simulink model "APP_SelSig"  (R2018a)
settings: configuration reference "cs_ert" (kept outside this file)
model workspace (MAT data in the model file):
  APP_SelSig_DT = 10
values from neighbouring files (symbols this model uses):
  APP_duLimErrPos_C = 1000.0    [APP_SelSig.sldd]
  APP_uAPPDef_C = 0.0    [APP_SelSig.sldd]
  APP_uRaw2Offset_C = 0.0    [APP_SelSig.sldd]
  MoFAPP_dRawSigFac_C = 2.0    [APP_SelSig.sldd]
libraries: simulink x1, sllib x1
settings Model: DataDictionary=APP_SelSig.sldd  Creator=zhoutinglin  LastModifiedBy=zhoutinglin

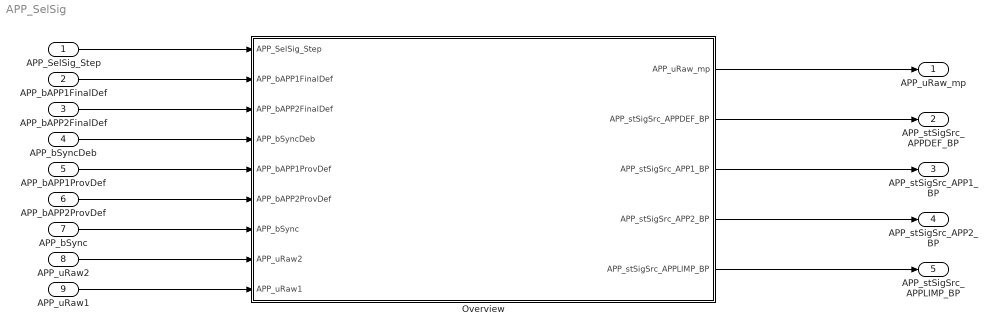
== system APP_SelSig ==
  APP_SelSig_Step : Inport  OutputFunctionCall=on
  APP_bAPP1FinalDef : Inport  Description=Status Sensor 1 of the acceleration pedal finally defect  Port=2  OutMin=0  OutMax=1  OutDataTypeStr=boolean  PortDimensions=[1 1]
  APP_bAPP2FinalDef : Inport  Description=Status Sensor 2 of the acceleration pedal finally defect  Port=3  OutMin=0  OutMax=1  OutDataTypeStr=boolean  PortDimensions=[1 1]
  APP_bSyncDeb : Inport  Description=Status debounced sync check  Port=4  OutMin=0  OutMax=1  OutDataTypeStr=boolean  PortDimensions=[1 1]
  APP_bAPP1ProvDef : Inport  Description=Status Sensor 1 of the acceleration pedal temporary defect  Port=5  OutMin=0  OutMax=1  OutDataTypeStr=boolean  PortDimensions=[1 1]
  APP_bAPP2ProvDef : Inport  Description=Status Sensor 2 of the acceleration pedal temporary defect  Port=6  OutMin=0  OutMax=1  OutDataTypeStr=boolean  PortDimensions=[1 1]
  APP_bSync : Inport  Description=Status temporary sync check  Port=7  OutMin=0  OutMax=1  OutDataTypeStr=boolean  PortDimensions=[1 1]
  APP_uRaw2 : Inport  Description=Acceleration Pedal Position E  Port=8  OutMin=0  OutMax=5000  OutDataTypeStr=Volt_mV  Unit=mv  PortDimensions=[1 1]
  APP_uRaw1 : Inport  Description=Acceleration Pedal Position D  Port=9  OutMin=0  OutMax=5000  OutDataTypeStr=Volt_mV  Unit=mv  PortDimensions=[1 1]
  Overview : Subsystem
  APP_uRaw_mp : Outport  Description=Acceleration pedal position raw value  OutMin=0  OutMax=5000  OutDataTypeStr=Volt_mV  Unit=mv  PortDimensions=[1 1]
  APP_stSigSrc_APPDEF_BP : Outport  Description=both the sensors are defective. Use the default value  Port=2  OutMin=0  OutMax=1  OutDataTypeStr=boolean  PortDimensions=[1 1]
  APP_stSigSrc_APP1_BP : Outport  Description=Sensor 1 is the reference variable, Sensor 2 value is defective  Port=3  OutMin=0  OutMax=1  OutDataTypeStr=boolean  PortDimensions=[1 1]
  APP_stSigSrc_APP2_BP : Outport  Description=Sensor 2 is the reference variable,Sensor1 value is defective  Port=4  OutMin=0  OutMax=1  OutDataTypeStr=boolean  PortDimensions=[1 1]
  APP_stSigSrc_APPLIMP_BP : Outport  Description=Substitute operation active, accelerator pedal sensor value and accelerator pedal sensor increase are limited  Port=5  OutMin=0  OutMax=1  OutDataTypeStr=boolean  PortDimensions=[1 1]
  wires:
  APP_SelSig_Step/1 -> Overview/1(APP_SelSig_Step)
  APP_bAPP1FinalDef/1 -> Overview/2(APP_bAPP1FinalDef)
  APP_bAPP2FinalDef/1 -> Overview/3(APP_bAPP2FinalDef)
  APP_bSyncDeb/1 -> Overview/4(APP_bSyncDeb)
  APP_bAPP1ProvDef/1 -> Overview/5(APP_bAPP1ProvDef)
  APP_bAPP2ProvDef/1 -> Overview/6(APP_bAPP2ProvDef)
  APP_bSync/1 -> Overview/7(APP_bSync)
  APP_uRaw2/1 -> Overview/8(APP_uRaw2)
  APP_uRaw1/1 -> Overview/9(APP_uRaw1)
  Overview/1(APP_uRaw_mp) -> APP_uRaw_mp/1
  Overview/2(APP_stSigSrc_APPDEF_BP) -> APP_stSigSrc_APPDEF_BP/1
  Overview/3(APP_stSigSrc_APP1_BP) -> APP_stSigSrc_APP1_BP/1
  Overview/4(APP_stSigSrc_APP2_BP) -> APP_stSigSrc_APP2_BP/1
  Overview/5(APP_stSigSrc_APPLIMP_BP) -> APP_stSigSrc_APPLIMP_BP/1

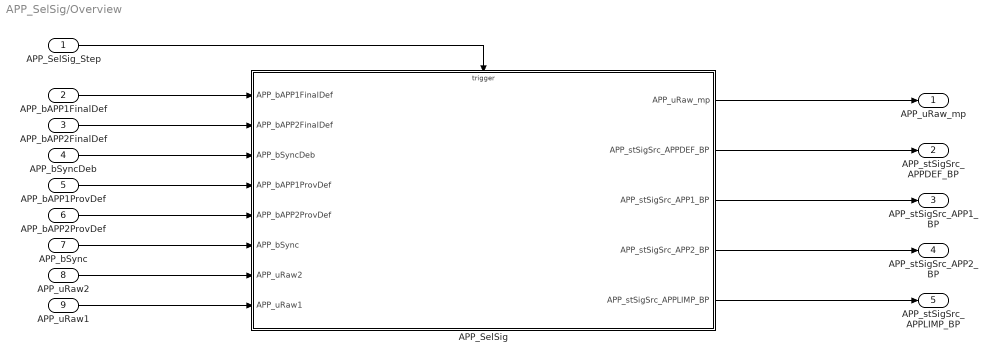
== system APP_SelSig/Overview ==
  APP_SelSig_Step : Inport
  APP_bAPP1FinalDef : Inport  Port=2
  APP_bAPP2FinalDef : Inport  Port=3
  APP_bSyncDeb : Inport  Port=4
  APP_bAPP1ProvDef : Inport  Port=5
  APP_bAPP2ProvDef : Inport  Port=6
  APP_bSync : Inport  Port=7
  APP_uRaw2 : Inport  Port=8
  APP_uRaw1 : Inport  Port=9
  APP_SelSig : Subsystem
  APP_uRaw_mp : Outport
  APP_stSigSrc_APPDEF_BP : Outport  Port=2
  APP_stSigSrc_APP1_BP : Outport  Port=3
  APP_stSigSrc_APP2_BP : Outport  Port=4
  APP_stSigSrc_APPLIMP_BP : Outport  Port=5
  wires:
  APP_bAPP1FinalDef/1 -> APP_SelSig/1(APP_bAPP1FinalDef)
  APP_bAPP2FinalDef/1 -> APP_SelSig/2(APP_bAPP2FinalDef)
  APP_bSyncDeb/1 -> APP_SelSig/3(APP_bSyncDeb)
  APP_bAPP1ProvDef/1 -> APP_SelSig/4(APP_bAPP1ProvDef)
  APP_bAPP2ProvDef/1 -> APP_SelSig/5(APP_bAPP2ProvDef)
  APP_bSync/1 -> APP_SelSig/6(APP_bSync)
  APP_uRaw2/1 -> APP_SelSig/7(APP_uRaw2)
  APP_uRaw1/1 -> APP_SelSig/8(APP_uRaw1)
  APP_SelSig/1(APP_uRaw_mp) -> APP_uRaw_mp/1
  APP_SelSig/2(APP_stSigSrc_APPDEF_BP) -> APP_stSigSrc_APPDEF_BP/1
  APP_SelSig/3(APP_stSigSrc_APP1_BP) -> APP_stSigSrc_APP1_BP/1
  APP_SelSig/4(APP_stSigSrc_APP2_BP) -> APP_stSigSrc_APP2_BP/1
  APP_SelSig/5(APP_stSigSrc_APPLIMP_BP) -> APP_stSigSrc_APPLIMP_BP/1
  APP_SelSig_Step/1 -> APP_SelSig/Trigger

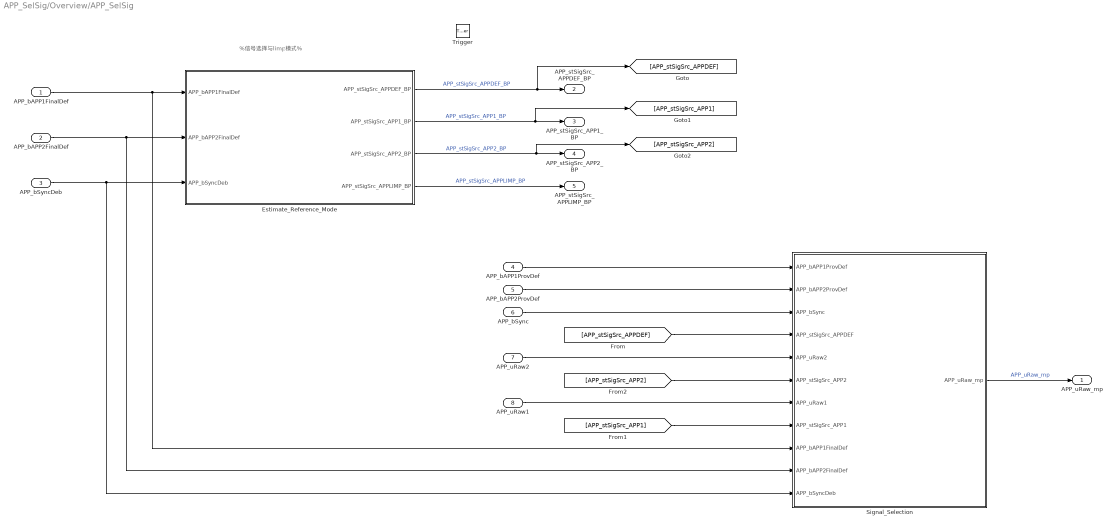
== system APP_SelSig/Overview/APP_SelSig ==
  note: %信号选择与limp模式%
  APP_bAPP1FinalDef : Inport
  APP_bAPP2FinalDef : Inport  Port=2
  APP_bSyncDeb : Inport  Port=3
  APP_bAPP1ProvDef : Inport  Port=4
  APP_bAPP2ProvDef : Inport  Port=5
  APP_bSync : Inport  Port=6
  APP_uRaw2 : Inport  Tag=mv  Port=7
  APP_uRaw1 : Inport  Tag=mv  Port=8
  Trigger : TriggerPort  TriggerType=function-call  VariantControl=Variant  PortDimensions=1
  Estimate_Reference_Mode : Subsystem
  Signal_Selection : Subsystem
  APP_uRaw_mp : Outport  Tag=mv
  APP_stSigSrc_APPDEF_BP : Outport  Port=2
  APP_stSigSrc_APP1_BP : Outport  Port=3
  APP_stSigSrc_APP2_BP : Outport  Port=4
  APP_stSigSrc_APPLIMP_BP : Outport  Port=5
  wires:
  APP_bAPP1FinalDef/1 -> Signal_Selection/9(APP_bAPP1FinalDef), Estimate_Reference_Mode/1(APP_bAPP1FinalDef)
  APP_bAPP2ProvDef/1 -> Signal_Selection/2(APP_bAPP2ProvDef)
  Signal_Selection/1(APP_uRaw_mp) -> APP_uRaw_mp/1  "APP_uRaw_mp"
  [APP_stSigSrc_APPDEF] -> Signal_Selection/4(APP_stSigSrc_APPDEF)
  [APP_stSigSrc_APP2] -> Signal_Selection/6(APP_stSigSrc_APP2)
  [APP_stSigSrc_APP1] -> Signal_Selection/8(APP_stSigSrc_APP1)
  Estimate_Reference_Mode/4(APP_stSigSrc_APPLIMP_BP) -> APP_stSigSrc_APPLIMP_BP/1  "APP_stSigSrc_APPLIMP_BP"
  Estimate_Reference_Mode/2(APP_stSigSrc_APP1_BP) -> [APP_stSigSrc_APP1], APP_stSigSrc_APP1_BP/1  "APP_stSigSrc_APP1_BP"
  APP_bAPP2FinalDef/1 -> Signal_Selection/10(APP_bAPP2FinalDef), Estimate_Reference_Mode/2(APP_bAPP2FinalDef)
  APP_uRaw1/1 -> Signal_Selection/7(APP_uRaw1)
  Estimate_Reference_Mode/3(APP_stSigSrc_APP2_BP) -> APP_stSigSrc_APP2_BP/1, [APP_stSigSrc_APP2]  "APP_stSigSrc_APP2_BP"
  APP_bAPP1ProvDef/1 -> Signal_Selection/1(APP_bAPP1ProvDef)
  APP_bSyncDeb/1 -> Signal_Selection/11(APP_bSyncDeb), Estimate_Reference_Mode/3(APP_bSyncDeb)
  Estimate_Reference_Mode/1(APP_stSigSrc_APPDEF_BP) -> [APP_stSigSrc_APPDEF], APP_stSigSrc_APPDEF_BP/1  "APP_stSigSrc_APPDEF_BP"
  APP_bSync/1 -> Signal_Selection/3(APP_bSync)
  APP_uRaw2/1 -> Signal_Selection/5(APP_uRaw2)

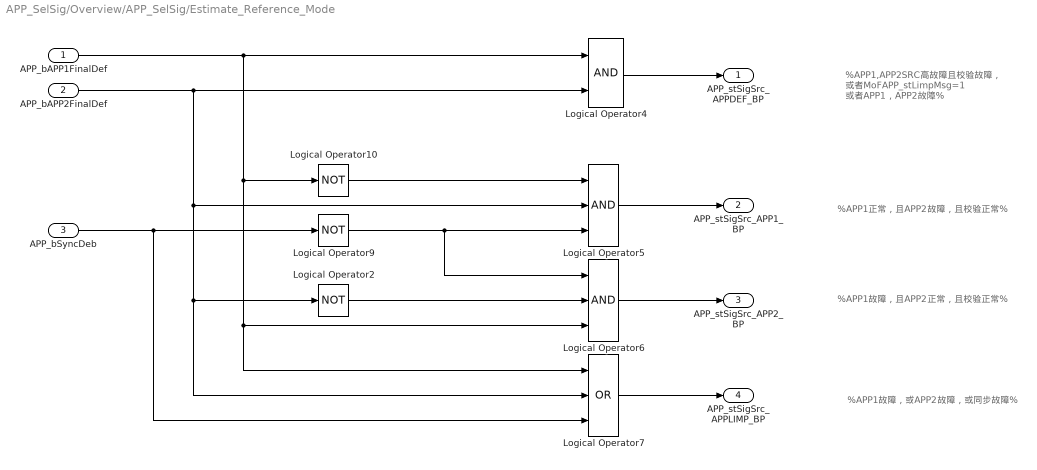
== system APP_SelSig/Overview/APP_SelSig/Estimate_Reference_Mode ==
  note: %APP1正常，且APP2故障，且校验正常%
  note: %APP1故障，且APP2正常，且校验正常%
  note: %APP1故障，或APP2故障，或同步故障%
  note: %APP1,APP2SRC高故障且校验故障，
      | 或者MoFAPP_stLimpMsg=1
      | 或者APP1，APP2故障%
  APP_bAPP1FinalDef : Inport
  APP_bAPP2FinalDef : Inport  Port=2
  APP_bSyncDeb : Inport  Port=3
  Logical Operator10 : Logic  Operator=NOT  AllPortsSameDT=off  OutDataTypeStr=boolean
  Logical Operator2 : Logic  Operator=NOT  AllPortsSameDT=off  OutDataTypeStr=boolean
  Logical Operator4 : Logic  OutDataTypeStr=boolean
  Logical Operator5 : Logic  Inputs=3  OutDataTypeStr=boolean
  Logical Operator6 : Logic  Inputs=3  OutDataTypeStr=boolean
  Logical Operator7 : Logic  Operator=OR  Inputs=3  OutDataTypeStr=boolean
  Logical Operator9 : Logic  Operator=NOT  AllPortsSameDT=off  OutDataTypeStr=boolean
  APP_stSigSrc_APPDEF_BP : Outport
  APP_stSigSrc_APP1_BP : Outport  Port=2
  APP_stSigSrc_APP2_BP : Outport  Port=3
  APP_stSigSrc_APPLIMP_BP : Outport  Port=4
  wires:
  Logical Operator2/1 -> Logical Operator6/2
  Logical Operator9/1 -> Logical Operator5/3, Logical Operator6/1
  Logical Operator10/1 -> Logical Operator5/1
  APP_bSyncDeb/1 -> Logical Operator9/1, Logical Operator7/3
  APP_bAPP2FinalDef/1 -> Logical Operator4/2, Logical Operator7/2, Logical Operator2/1, Logical Operator5/2
  APP_bAPP1FinalDef/1 -> Logical Operator4/1, Logical Operator10/1, Logical Operator7/1, Logical Operator6/3
  Logical Operator7/1 -> APP_stSigSrc_APPLIMP_BP/1
  Logical Operator6/1 -> APP_stSigSrc_APP2_BP/1
  Logical Operator5/1 -> APP_stSigSrc_APP1_BP/1
  Logical Operator4/1 -> APP_stSigSrc_APPDEF_BP/1

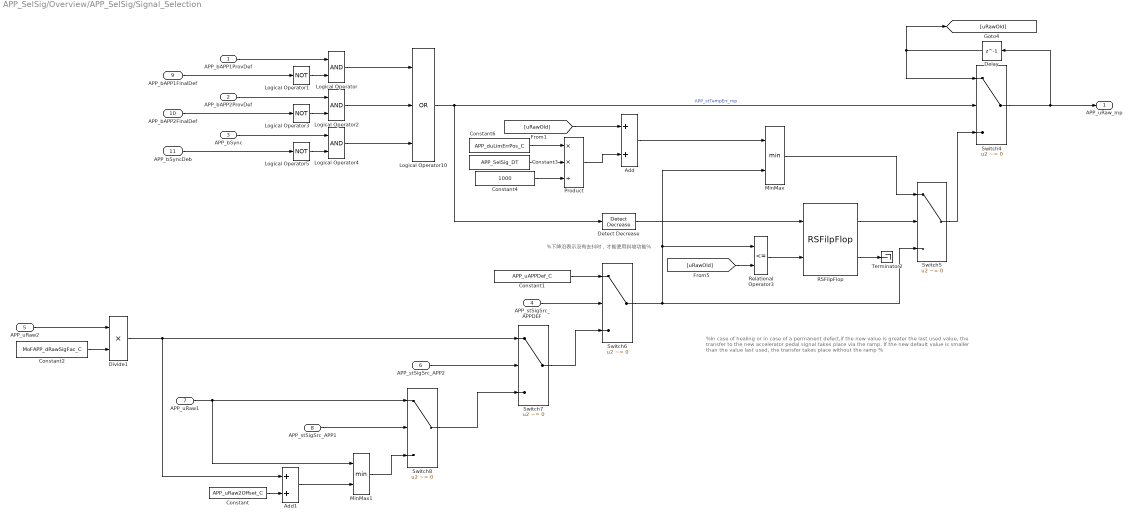
== system APP_SelSig/Overview/APP_SelSig/Signal_Selection ==
  note: %下降沿表示没有去抖时，才能使用斜坡功能%
  note: %In case of healing or in case of a permanent defect,if the new value is greater the last used value,
      | the transfer to the new accelerator pedal signal takes place via the ramp. If the new default value
      | is smaller than the value last used, the transfer takes place without the ramp %
  APP_bAPP1ProvDef : Inport  Tag=-
  APP_bAPP2ProvDef : Inport  Tag=-  Port=2
  APP_bSync : Inport  Tag=-  Port=3
  APP_stSigSrc_APPDEF : Inport  Port=4
  APP_uRaw2 : Inport  Tag=mv  Port=5
  APP_stSigSrc_APP2 : Inport  Port=6
  APP_uRaw1 : Inport  Tag=mv  Port=7
  APP_stSigSrc_APP1 : Inport  Port=8
  APP_bAPP1FinalDef : Inport  Port=9
  APP_bAPP2FinalDef : Inport  Port=10
  APP_bSyncDeb : Inport  Port=11
  Add : Sum  InputSameDT=on
  Add1 : Sum  InputSameDT=on
  Constant : Constant  Value=APP_uRaw2Offset_C
  Constant1 : Constant  Value=APP_uAPPDef_C
  Constant2 : Constant  Value=MoFAPP_dRawSigFac_C  SampleTime=-1
  Constant3 : Constant  Value=APP_SelSig_DT  OutDataTypeStr=Inherit: Inherit via back propagation
  Constant4 : Constant  Value=1000  OutDataTypeStr=int16
  Constant6 : Constant  Value=APP_duLimErrPos_C
  Delay : Delay  DelayLength=1  InitialCondition=0
  Detect Decrease : simulink/Logic and Bit Operations/Detect Decrease  vinit=0.0  OutDataTypeStr=boolean
  Divide1 : Product  Inputs=**  OutDataTypeStr=Inherit: Inherit via back propagation
  Logical Operator : Logic  OutDataTypeStr=boolean
  Logical Operator1 : Logic  Operator=NOT  AllPortsSameDT=off  OutDataTypeStr=boolean
  Logical Operator10 : Logic  Operator=OR  Inputs=3  OutDataTypeStr=boolean
  Logical Operator2 : Logic  OutDataTypeStr=boolean
  Logical Operator3 : Logic  Operator=NOT  AllPortsSameDT=off  OutDataTypeStr=boolean
  Logical Operator4 : Logic  OutDataTypeStr=boolean
  Logical Operator5 : Logic  Operator=NOT  AllPortsSameDT=off  OutDataTypeStr=boolean
  MinMax : MinMax  Inputs=2
  MinMax1 : MinMax  Inputs=2  InputSameDT=on
  Product : Product  Inputs=**/  OutDataTypeStr=Inherit: Inherit via back propagation
  RSFilpFlop : sllib/RSFilpFlop
      settings: SourceProductName=sllib
  Relational Operator3 : RelationalOperator  Operator=<=  OutDataTypeStr=boolean  RndMeth=Nearest  InputSameDT=on
  Switch{4..8} (5 alike) : Switch  Criteria=u2 ~= 0  InputSameDT=on
  Terminator2 : Terminator
  APP_uRaw_mp : Outport  Tag=mv
  wires:
  APP_bAPP1FinalDef/1 -> Logical Operator1/1
  APP_bAPP2FinalDef/1 -> Logical Operator3/1
  APP_bSyncDeb/1 -> Logical Operator5/1
  Divide1/1 -> Switch7/1, Add1/1
  Constant/1 -> Add1/2
  APP_uRaw1/1 -> Switch8/1, MinMax1/1
  APP_stSigSrc_APP2/1 -> Switch7/2
  Switch8/1 -> Switch7/3
  APP_uRaw2/1 -> Divide1/1
  Constant1/1 -> Switch6/1
  Add1/1 -> MinMax1/2
  APP_stSigSrc_APP1/1 -> Switch8/2
  APP_stSigSrc_APPDEF/1 -> Switch6/2
  MinMax1/1 -> Switch8/3
  Switch7/1 -> Switch6/3
  Constant2/1 -> Divide1/2
  Detect Decrease/1 -> RSFilpFlop/1
  Relational Operator3/1 -> RSFilpFlop/2
  Switch4/1 -> APP_uRaw_mp/1, Delay/1
  Delay/1 -> Switch4/1, [uRawOld]
  RSFilpFlop/1 -> Switch5/2
  Switch5/1 -> Switch4/3
  RSFilpFlop/2 -> Terminator2/1
  Logical Operator10/1 -> Detect Decrease/1, Switch4/2  "APP_stTempErr_mp"
  APP_bAPP1ProvDef/1 -> Logical Operator/1
  Logical Operator1/1 -> Logical Operator/2
  APP_bAPP2ProvDef/1 -> Logical Operator2/1
  Logical Operator3/1 -> Logical Operator2/2
  Logical Operator5/1 -> Logical Operator4/2
  Logical Operator/1 -> Logical Operator10/1
  Logical Operator2/1 -> Logical Operator10/2
  Logical Operator4/1 -> Logical Operator10/3
  APP_bSync/1 -> Logical Operator4/1
  [uRawOld] -> Relational Operator3/2
  Switch6/1 -> Switch5/3, Relational Operator3/1, MinMax/2
  [uRawOld] -> Add/1
  Add/1 -> MinMax/1
  MinMax/1 -> Switch5/1
  Product/1 -> Add/2
  Constant6/1 -> Product/1
  Constant3/1 -> Product/2
  Constant4/1 -> Product/3
